simulink model "TPTC_Vehicle_dynamics_pedal2torque_NeglectSOC_R2024b"  (R2024b)
settings: Solver=ode23tb  StartTime=0.0  StopTime=40  RelTol=1e-3
model workspace (MAT data in the model file):
  BattChrgMax = -500000
  BattDischrgMax = 500000
  ChrgLmt_bpt = [1 1 1 1 1 1 1 1 0.7 0.35 0]
  DischrgLmt_bpt = [0 0.35 0.7 1 1 1 1 1 1 1 1]
  SOC_bpt = [0 10 20 30 40 50 60 70 80 90 100]
  motorMaxTorqueNm = [500 500 500 500 500 500 416.666666667 357.142857143 312.5 277.777777778 250 227.272727273 208.333333333 192.307692308 178.571428571 166.666666667]
  motorSpeedRadPs = [0 40 80 120 160 200 240 280 320 360 400 440 480 520 560 600]
undefined symbols (not defined in the file or in its folder): alpha_thr, dspblkCoreblockFVToolHelper, eta_drv, gcbh, gear_ratio_F, gear_ratio_R, J_axle, Kd_damp, R_tire, T_active, T_damp_lim, tau_lpf_damp, Tlim_down_rate, Tlim_up_rate, Tmax_mot, Ts_asr
libraries: autolibsharedcoupling x8, simulink x3, autolibshareddiff x2, autolibmappedmotor x2, slpidlib x1, autolibdatasheetbattery x1, sim3dlib x1, sim3dautolib x1, vehdynlibsteering x1
(part 1 of 3)
settings Model: Creator=jchu  LastModifiedBy=woaiw
settings ConfigComp: CovBoundaryAbsTol=1.0e-5

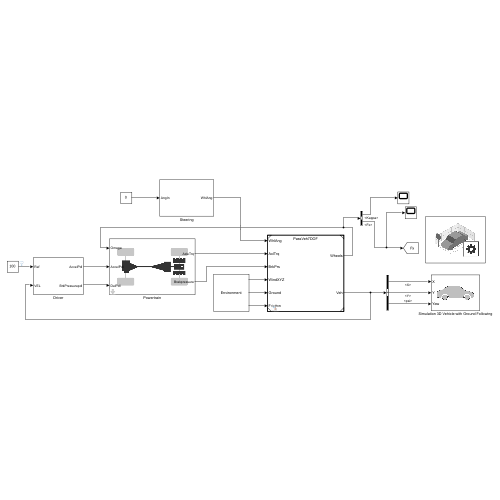
[thumbnail: Simulink's stored preview of the top-level diagram]
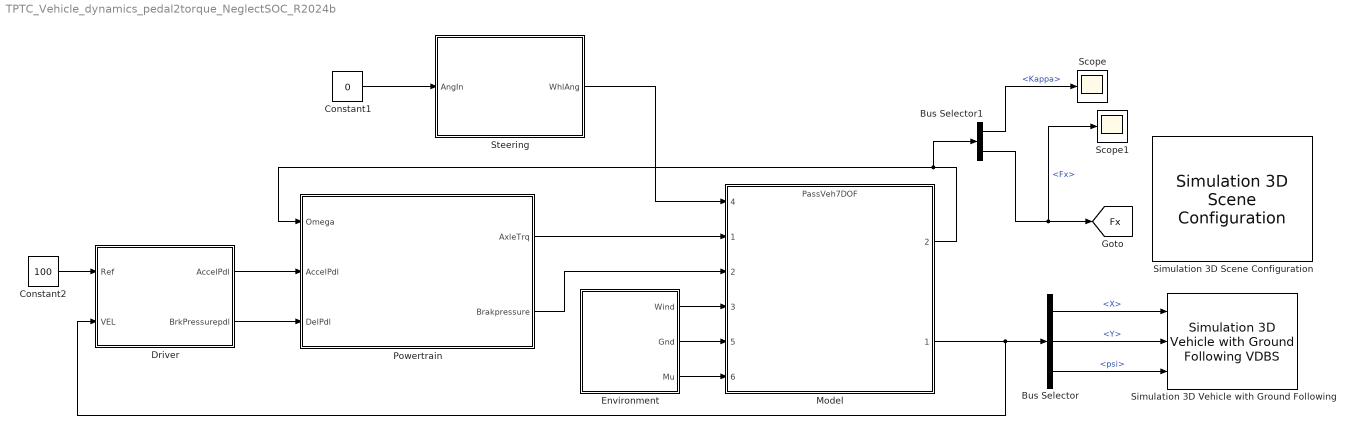
== system TPTC_Vehicle_dynamics_pedal2torque_NeglectSOC_R2024b ==
  Bus Selector : BusSelector  OutputSignals=InertFrm.Cg.Disp.X,InertFrm.Cg.Disp.Y,InertFrm.Cg.Ang.psi
  Bus Selector1 : BusSelector  OutputSignals=TireFrame.Kappa,TireFrame.Fx
  Constant1 : Constant  Value=0
  Constant2 : Constant  Value=100
  Driver : Subsystem
  Environment : Subsystem
      mask Display: disp('Environment')
  Model : ModelReference  ModelNameDialog=PassVeh7DOF.slx  SimulationMode=Normal  ModelReferenceVersion=9.3
      settings: PortSchema="{\"entries\":[{\"content\":{\"sides\":[{\"content\":{\"connectorIds\":[\"In4\",\"In1\",\"In2\",\"In3\",\"In5\",\"In6\"]},\"type\":\"ConnectorPlacement.EquallySpacedRectSide\",\"uuid\":\"e9709a47-3cb3-4a3a-94dc-e137fda36ac7\"},{\"content\":{\"connectorIds\":[\"Out2\",\"Out1\"],\"side\":\"RIGHT\"},\"type\":\"ConnectorPlacement.EquallySpacedRectSide\",\"uuid\":\"17c9465a-c7d2-47f9-932e-b722968c60f5\"},{\"content\":{\"side\":\"TOP\"},\"type\":\"ConnectorPlacement.EquallySpacedRectSide\",\"uuid\":\"38cd0d31-1510-4d7f-a224-4b6e7eb516ec\"}]},\"type\":\"ConnectorPlacement.EquallySpacedConnector\",\"uuid\":\"ef4f9ae8-cb52-4422-b25b-7a352d7601ce\"}],\"packageUris\":[\"http://schema.mathworks.com/mf0/Connector/R2020b\"],\"version\":\"1.0\"}"
  Powertrain : Subsystem
      mask DialogControl ParameterGroupVar Prompt: 参数
      mask Display: image('vdbslibpt.png');
  Scope : Scope
  Scope1 : Scope
  Simulation 3D Scene Configuration : sim3dlib/Simulation 3D Scene Configuration  Priority=0  ProjectFormat=Default Scenes  SceneDesc=Straight road  ProjectName=D:\Program Files\MATLAB\R2026a\toolbox\shared\sim3d_projects\automotive_project_windows\UE\WindowsNoEditor\VehicleSimulation.exe  ScenePath=/Game/Maps/HwStrght  EnableOpenDRIVE=off  vehTagList={'Custom';'Scene Origin';'SimulinkVehicle1'}  vehTag=SimulinkVehicle1  FreeCameraDefaultInitialTranslation=[-6, 0, 2]  FreeCameraDefaultInitialRotation=[0, -15, 0]  FreeCameraInitialTranslation=[0, 0, 0]  FreeCameraInitialRotation=[0, 0, 0]  OpVisEn=off  Ts=.02  EnableWindow=on  EnableRemoteAccess=off  SimulationMode=CoSimulation  SimulateUsing=Interpreted execution  EnableAnimationRecording=off  OverrideDefaultRecording=off  AnimationRecordingFileName=sim3dAnimation.mat  AnimationRecordingInterval=[0 inf]  EnableWeather=off  SunAzimuth=90  SunAltitude=40.0  EnableGeospatialSun=off  Latitude=0  Longitude=0  Date=2023-01-01  Time=10:30:00  GeoTimeZone=-5.0  SunDaylightSaving=off  wind=1  clouds=10  EnableVolumetricClouds=off  CloudCoverage=0  CloudAltitude=6  fog=0  rain=0  RaindropsEffect=off  SnowDensity=0  EnableGeospatial=off  UseTrueOrigin=off  OriginHeight=200  OriginLatitude=40.744652  OriginLongitude=-73.988864  MapStyle=Aerial  AdditionalAssetIDs=[]  UseAdvancedSunSky=off  SolarTime=11  TimeZone=-5  Day=21  Month=9  Year=2022  UseDaylightSavingTime=on  DSTStartDay=10  DSTStartMonth=3  DSTEndDay=3  DSTEndMonth=11  DSTSwitchHour=2  sensorTag=MainCamera1  sensorId=1  sensorName=MainCamera1  mountLoc=Origin  offsetFlag=off  tmountOffset=[0, 0, 0]  rmountOffset=[0, 0, 0]  HorizontalResolution=1280  VerticalResolution=720  HorizontalFOV=60  mountPoint=[0 0 0]  mountOrientation=[0 0 0]  aMode=2  ID=1  GeoTrigger=Inactive
      settings: LibrarySourceBlock=vehdynlibsim3dcore/Simulation 3D Scene Configuration
  Simulation 3D Vehicle with Ground Following : sim3dautolib/Simulation 3D Vehicle with Ground Following VDBS  Priority=-1  PassVehMesh=Muscle car  MeshPath=/MathWorksSimulation/Vehicles/Muscle/Meshes/SK_MuscleCar.SK_MuscleCar  TrackWidth=1.9  WheelBase=3  WheelRadius=0.35  VehColor=Red  InitialPos=[0, 0, 0]  InitialRot=[0, 0, 0]  ActorName=SimulinkVehicle1  VehLightsControl=off  HeadlightColor=[ 1, 1, 1 ]  HighBeamIntensity=100000  LowBeamIntensity=60000  HighBeamConeAngle=1.22  LowBeamConeAngle=1.22  LeftHeadlightOrientation=[ 0, 0 ]  RightHeadlightOrientation=[ 0, 0 ]  BrakelightIntensity=200  ReverselightIntensity=500  SignallightIntensity=500  SignallightPeriod=1  SignalPulseWidth=50  SampleTime=-1  ActorType=SimulinkVehicle  ID=1  aMode=2  ActorTag=SimulinkVehicle1  CoordinateScheme=SAE
      settings: LibrarySourceBlock=vehdynlibsim3d/Simulation 3D Vehicle with Ground Following
  Steering : Subsystem
  tag scope: Fx=global
  wires:
  Bus Selector/2 -> Simulation 3D Vehicle with Ground Following/2  "<Y>"
  Bus Selector/1 -> Simulation 3D Vehicle with Ground Following/1  "<X>"
  Bus Selector/3 -> Simulation 3D Vehicle with Ground Following/3  "<psi>"
  Environment/1(Wind) -> Model/3
  Environment/2(Gnd) -> Model/5
  Environment/3(Mu) -> Model/6
  Constant1/1 -> Steering/1(AngIn)
  Steering/1(WhlAng) -> Model/4
  Model/2 -> Bus Selector1/1, Powertrain/1(Omega)
  Powertrain/2(Brakpressure) -> Model/2
  Constant2/1 -> Driver/1(Ref)
  Model/1 -> Driver/2(VEL), Bus Selector/1
  Driver/1(AccelPdl) -> Powertrain/2(AccelPdl)
  Driver/2(BrkPressurepdl) -> Powertrain/3(DelPdl)
  Powertrain/1(AxleTrq) -> Model/1
  Bus Selector1/1 -> Scope/1  "<Kappa>"
  Bus Selector1/2 -> Scope1/1, [Fx]  "<Fx>"

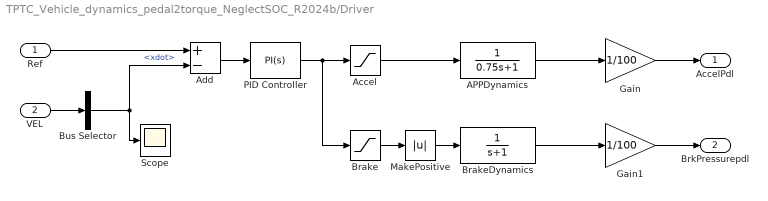
== system TPTC_Vehicle_dynamics_pedal2torque_NeglectSOC_R2024b/Driver ==
  Ref : Inport
  VEL : Inport  Port=2
  APPDynamics : TransferFcn  Denominator=[0.75 1]
  Accel : Saturate  UpperLimit=100  LowerLimit=0
  Add : Sum  Inputs=+-
  Brake : Saturate  UpperLimit=0  LowerLimit=-100
  BrakeDynamics : TransferFcn  Denominator=[1 1]
  Bus Selector : BusSelector  OutputSignals=BdyFrm.Cg.Vel.xdot
  Gain : Gain  Gain=1/100
  Gain1 : Gain  Gain=1/100
  MakePositive : Abs  SaturateOnIntegerOverflow=off
  PID Controller : slpidlib/PID Controller  Controller=PI  Form=Parallel  TimeDomain=Continuous-time  UseExternalTs=off  SampleTime=-1  IntegratorMethod=Forward Euler  FilterMethod=Forward Euler  ControllerParametersSource=internal  P=20  I=1  UseKiTs=off  D=0  UseExternalDerivativeSource=off  N=100  UseFilter=on  TunerSelectOption=Transfer Function Based (PID Tuner App)  InitialConditionSource=internal  InitialConditionForIntegrator=0  InitialConditionForFilter=0  DifferentiatorICPrevScaledInput=0  ExternalReset=none  TrackingMode=off  Kt=1  LimitOutput=on  SatLimitsSource=internal  UpperSaturationLimit=100  LowerSaturationLimit=-100  LinearizeAsGain=on  AntiWindupMode=none  Kb=1  LimitIntegrator=off  UpperIntegratorSaturationLimit=inf  LowerIntegratorSaturationLimit=-inf  POutMin=[]  POutMax=[]  IOutMin=[]  IOutMax=[]  DOutMin=[]  DOutMax=[]  NOutMin=[]  NOutMax=[]  SumOutMin=[]  SumOutMax=[]  SaturationOutMin=[]  SaturationOutMax=[]  PParamMin=[]  PParamMax=[]  IParamMin=[]  IParamMax=[]  DParamMin=[]  DParamMax=[]  NParamMin=[]  NParamMax=[]  KbParamMin=[]  KbParamMax=[]  KtParamMin=[]  KtParamMax=[]  KbOutMin=[]  KbOutMax=[]  KtOutMin=[]  KtOutMax=[]  IntegratorOutMin=[]  IntegratorOutMax=[]  FilterOutMin=[]  FilterOutMax=[]  SumI1OutMin=[]  SumI1OutMax=[]  SumI2OutMin=[]  SumI2OutMax=[]  SumI3OutMin=[]  SumI3OutMax=[]  SumI4OutMin=[]  SumI4OutMax=[]  SumDOutMin=[]  SumDOutMax=[]  DifferentiatorOutMin=[]  DifferentiatorOutMax=[]  FilterDiffOutCoefMin=[]  FilterDiffOutCoefMax=[]  ReciprocalOutMin=[]  ReciprocalOutMax=[]  SumDenOutMin=[]  SumDenOutMax=[]  SumNumOutMin=[]  SumNumOutMax=[]  DivideOutMin=[]  DivideOutMax=[]  UdiffTsProdOutMin=[]  UdiffTsProdOutMax=[]  NTsProdOutMin=[]  NTsProdOutMax=[]  UintegralTsProdOutMin=[]  UintegralTsProdOutMax=[]  UngainTsProdOutMin=[]  UngainTsProdOutMax=[]  ClampingZeroOutDataTypeStr=Inherit: Inherit via back propagation  ClampingZeroOutMin=[]  ClampingZeroOutMax=[]  FilterDenConstantOutDataTypeStr=Inherit: Inherit via back propagation  FilterDenConstantOutMin=[]  FilterDenConstantOutMax=[]  PCopyOutDataTypeStr=Inherit: Inherit via back propagation  PCopyOutMin=[]  PCopyOutMax=[]  NCopyOutDataTypeStr=Inherit: Inherit via back propagation  NCopyOutMin=[]  NCopyOutMax=[]  IntegratorContinuousStateAttributes=''  IntegratorStateMustResolveToSignalObject=off  IntegratorRTWStateStorageClass=Auto  FilterContinuousStateAttributes=''  FilterStateMustResolveToSignalObject=off  FilterRTWStateStorageClass=Auto  ParallelPVariant=InternalParameters  IdealPVariant=Disabled  IVariant=InternalParameters  DVariant=Disabled  IntegratorVariant=Continuous  SatVariant=Enabled  AWVariant=Passthrough  PCopyVariant=Disabled  TRVariant=Disabled  FdbkBlocksVariant=Forward  IdealPFdbkVariant=Disabled  SatFdbkVariant=Disabled  DerivativeFilterVariant=Disabled  NVariant=Disabled  NCopyVariant=Disabled_SignalSpec  FilterICVariant=Disabled  IntegratorICVariant=InternalICs  ExternalResetVariant=Disabled  TRSumVariant=Passthrough  SumFdbkVariant=Disabled  SumVariant=Sum_PI  TsampFilterVariant=InternalTs  TsampNgainVariant=Passthrough  TsampIntegralVariant=Disabled_SignalSpec  ExternalSaturationOutDataTypeStr=Inherit: Same as second input  DerivativeSourceVariant=Disabled  PreIntVariant=InternalPreInt
  Scope : Scope
  AccelPdl : Outport
  BrkPressurepdl : Outport  Port=2
  wires:
  APPDynamics/1 -> Gain/1
  PID Controller/1 -> Accel/1, Brake/1
  MakePositive/1 -> BrakeDynamics/1
  Accel/1 -> APPDynamics/1
  Add/1 -> PID Controller/1
  Brake/1 -> MakePositive/1
  Ref/1 -> Add/1
  BrakeDynamics/1 -> Gain1/1
  Gain/1 -> AccelPdl/1
  Gain1/1 -> BrkPressurepdl/1
  VEL/1 -> Bus Selector/1
  Bus Selector/1 -> Scope/1, Add/2  "<xdot>"

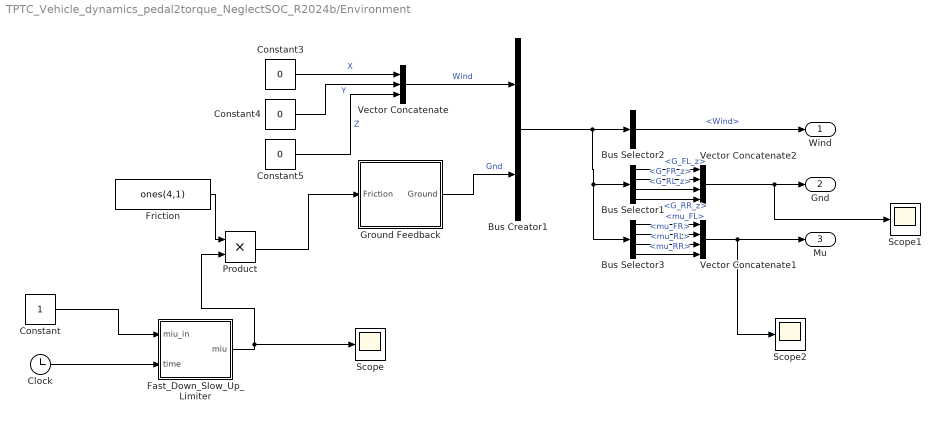
== system TPTC_Vehicle_dynamics_pedal2torque_NeglectSOC_R2024b/Environment ==
  Bus Creator1 : BusCreator  Inputs=2
  Bus Selector1 : BusSelector  OutputSignals=Gnd.z.G_FL_z,Gnd.z.G_FR_z,Gnd.z.G_RL_z,Gnd.z.G_RR_z
  Bus Selector2 : BusSelector  OutputSignals=Wind
  Bus Selector3 : BusSelector  OutputSignals=Gnd.mu.mu_FL,Gnd.mu.mu_FR,Gnd.mu.mu_RL,Gnd.mu.mu_RR
  Clock : Clock
  Constant : Constant
  Constant3 : Constant  Value=0
  Constant4 : Constant  Value=0
  Constant5 : Constant  Value=0
  Fast_Down_Slow_Up_Limiter : MATLAB Function  TreatAsAtomicUnit=on  SystemSampleTime=Ts_asr
  Friction : Constant  Value=ones(4,1)
  Ground Feedback : Subsystem  Variant=on  VariantControlMode=label  LabelModeActiveChoice=0
  Product : Product
  Scope : Scope
  Scope1 : Scope
  Scope2 : Scope
  Vector Concatenate : Concatenate  NumInputs=3
  Vector Concatenate1 : Concatenate  NumInputs=4
  Vector Concatenate2 : Concatenate  NumInputs=4
  Wind : Outport
  Gnd : Outport  Port=2
  Mu : Outport  Port=3
  wires:
  Constant5/1 -> Vector Concatenate/3  "Z"
  Vector Concatenate/1 -> Bus Creator1/1  "Wind"
  Constant3/1 -> Vector Concatenate/1  "X"
  Constant4/1 -> Vector Concatenate/2  "Y"
  Ground Feedback/1(Ground) -> Bus Creator1/2  "Gnd"
  Friction/1 -> Product/1
  Bus Selector3/1 -> Vector Concatenate1/1  "<mu_FL>"
  Vector Concatenate1/1 -> Scope2/1, Mu/1
  Bus Selector2/1 -> Wind/1  "<Wind>"
  Vector Concatenate2/1 -> Scope1/1, Gnd/1
  Bus Selector3/3 -> Vector Concatenate1/3  "<mu_RL>"
  Bus Selector3/4 -> Vector Concatenate1/4  "<mu_RR>"
  Bus Selector1/2 -> Vector Concatenate2/2  "<G_FR_z>"
  Bus Creator1/1 -> Bus Selector3/1, Bus Selector1/1, Bus Selector2/1
  Bus Selector3/2 -> Vector Concatenate1/2  "<mu_FR>"
  Bus Selector1/4 -> Vector Concatenate2/4  "<G_RR_z>"
  Bus Selector1/1 -> Vector Concatenate2/1  "<G_FL_z>"
  Bus Selector1/3 -> Vector Concatenate2/3  "<G_RL_z>"
  Product/1 -> Ground Feedback/1(Friction)
  Clock/1 -> Fast_Down_Slow_Up_Limiter/2(time)
  Constant/1 -> Fast_Down_Slow_Up_Limiter/1(miu_in)
  Fast_Down_Slow_Up_Limiter/1(miu) -> Product/2, Scope/1

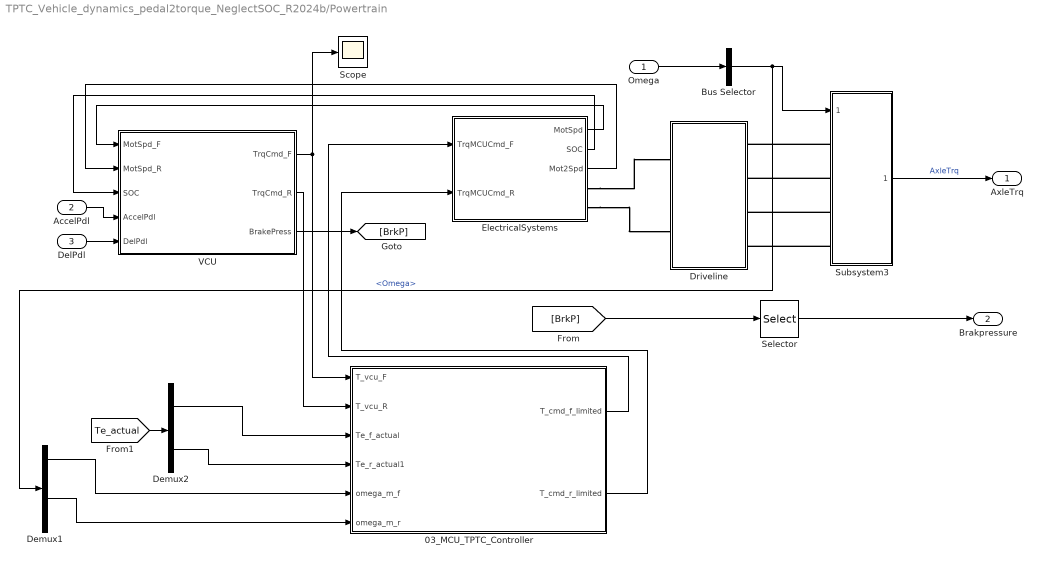
== system TPTC_Vehicle_dynamics_pedal2torque_NeglectSOC_R2024b/Powertrain ==
  Omega : Inport
  AccelPdl : Inport  Port=2
  DelPdl : Inport  Port=3
  03_MCU_TPTC_Controller : Subsystem
  Bus Selector : BusSelector  OutputSignals=TireFrame.Omega
  Demux1 : Demux
  Demux2 : Demux  Outputs=2
  Driveline : Subsystem
  ElectricalSystems : Subsystem
  Scope : Scope
  Selector : Selector  InputPortWidth=1  IndexOptions=Index vector (dialog)  Indices=[1 1 1 1]  OutputSizes=1
  Subsystem3 : Subsystem
  VCU : Subsystem
  AxleTrq : Outport
  Brakpressure : Outport  Port=2
  wires:
  ElectricalSystems/2(SOC) -> VCU/3(SOC)
  Subsystem3/1(AxleTrq) -> AxleTrq/1  "AxleTrq"
  AccelPdl/1 -> VCU/4(AccelPdl)
  Omega/1 -> Bus Selector/1
  Bus Selector/1 -> Demux1/1, Subsystem3/1(WhlSpd)  "<Omega>"
  ElectricalSystems/1(MotSpd) -> VCU/1(MotSpd_F)
  VCU/3(BrakePress) -> [BrkP]
  DelPdl/1 -> VCU/5(DelPdl)
  Selector/1 -> Brakpressure/1
  [BrkP] -> Selector/1
  VCU/1(TrqCmd_F) -> Scope/1, 03_MCU_TPTC_Controller/1(T_vcu_F)
  VCU/2(TrqCmd_R) -> 03_MCU_TPTC_Controller/2(T_vcu_R)
  03_MCU_TPTC_Controller/1("T_cmd_f_limited  ") -> ElectricalSystems/1(TrqMCUCmd_F)
  03_MCU_TPTC_Controller/2("T_cmd_r_limited ") -> ElectricalSystems/2(TrqMCUCmd_R)
  Demux1/3 -> 03_MCU_TPTC_Controller/6(omega_m_r)
  Demux1/1 -> 03_MCU_TPTC_Controller/5(omega_m_f)
  Demux2/1 -> 03_MCU_TPTC_Controller/3(Te_f_actual)
  Demux2/2 -> 03_MCU_TPTC_Controller/4(Te_r_actual1)
  ElectricalSystems/3(Mot2Spd) -> VCU/2(MotSpd_R)
  [Te_actual] -> Demux2/1
  connections:
  Subsystem3/LConn1 -- Driveline/RConn1
  ElectricalSystems/RConn1 -- Driveline/LConn1
  Subsystem3/LConn2 -- Driveline/RConn2
  Subsystem3/LConn3 -- Driveline/RConn3
  Subsystem3/LConn4 -- Driveline/RConn4
  ElectricalSystems/RConn2 -- Driveline/LConn2

== system TPTC_Vehicle_dynamics_pedal2torque_NeglectSOC_R2024b/Steering ==
  AngIn : Inport
  Ground1 : Ground
  Ground2 : Ground
  Kinematic Steering : vehdynlibsteering/Kinematic Steering  StrgType=Rack and pinion  StrgRatioType=Constant  Loc=Front  NrmlFctr=0.01  TrckWdth=1  WhlBase=1.524  Db=0  StrgRng=1.25*pi  StrgAngBpts="[-6.2832   -5.0265   -3.7699   -2.5133   -1.2566         0    1.2566    2.5133    3.7699    5.0265    6.2832]"  StrgRatioTbl=|  StrgRatio=100  PctAckIn=off  PctAck=100  PctAckTbl=ones(1,11)*100  StrgArmLngth=0.1  RckCsLngth=0.5  TieRodLngth=0.248  D=0.2  PnnRadius=0.00085818  PnnRadiusTbl="[0.0055    0.0055    0.0056    0.0057    0.0058    0.0057    0.0057    0.0057    0.0056    0.0055    0.0055]"  RodLngth=0.1  ParaArmLngth=0.9  aMode=2
      | [13.5000   13.3750   13.2500   13.1250   13.0000   13.0000   13.0000   13.1250   13.2500   13.3750   13.5000
      | ]
  Mux : Mux
  WhlAng : Outport
  wires:
  Kinematic Steering/3 -> Mux/2
  Ground1/1 -> Mux/3
  Ground2/1 -> Mux/4
  Kinematic Steering/2 -> Mux/1
  Mux/1 -> WhlAng/1
  AngIn/1 -> Kinematic Steering/1

== system TPTC_Vehicle_dynamics_pedal2torque_NeglectSOC_R2024b/Environment/Ground Feedback ==
  Friction : Inport
  Constant : Subsystem  VariantControl=0
  Ground : Outport  VectorParamsAs1DForOutWhenUnconnected=off

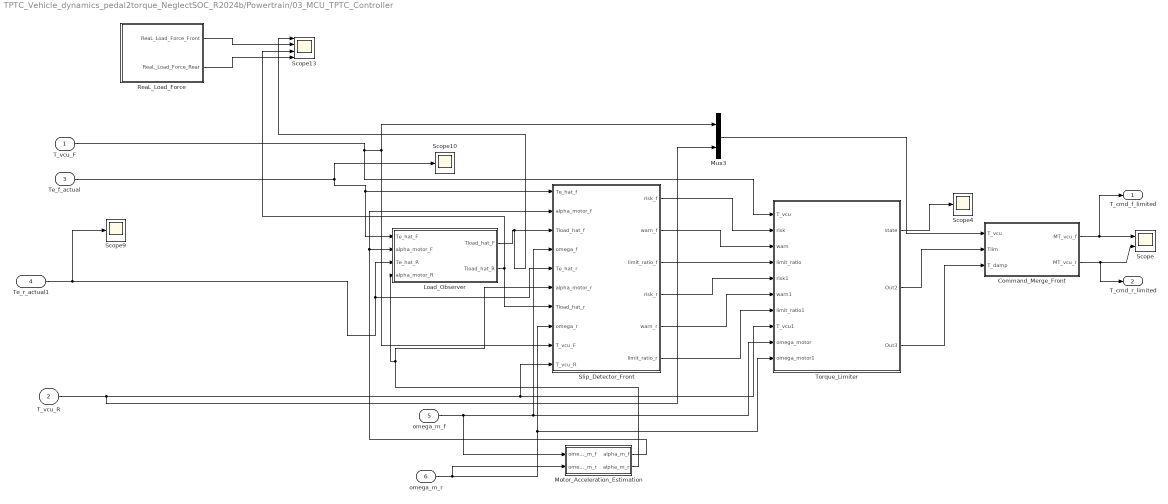
== system TPTC_Vehicle_dynamics_pedal2torque_NeglectSOC_R2024b/Powertrain/03_MCU_TPTC_Controller ==
  T_vcu_F : Inport
  T_vcu_R : Inport  Port=2
  Te_f_actual : Inport  Port=3
  Te_r_actual1 : Inport  Port=4
  omega_m_f : Inport  Port=5
  omega_m_r : Inport  Port=6
  Command_Merge_Front : Subsystem
  Load_Observer : Subsystem
  Motor_Acceleration_Estimation : Subsystem
  Mux3 : Mux  Inputs=2
  ReaL_Load_Force : Subsystem
  Scope : Scope  NumInputPorts=2
  Scope10 : Scope
  Scope13 : Scope  NumInputPorts=4
  Scope4 : Scope
  Scope9 : Scope
  Slip_Detector_Front : Subsystem
  Torque_Limiter : Subsystem
  "T_cmd_f_limited  " : Outport
  "T_cmd_r_limited " : Outport  Port=2
  wires:
  Motor_Acceleration_Estimation/2(alpha_m_r) -> Slip_Detector_Front/6(alpha_motor_r), Load_Observer/4(alpha_motor_R)
  Motor_Acceleration_Estimation/1(alpha_m_f) -> Slip_Detector_Front/2(alpha_motor_f), Load_Observer/2(alpha_motor_F)
  omega_m_r/1 -> Motor_Acceleration_Estimation/2(omega_m_r), Torque_Limiter/10(omega_motor1), Slip_Detector_Front/8(omega_r)
  Mux3/1 -> Command_Merge_Front/1(T_vcu)
  Command_Merge_Front/1(MT_vcu_f) -> "T_cmd_f_limited  "/1, Scope/1
  Command_Merge_Front/2(MT_vcu_r) -> Scope/2, "T_cmd_r_limited "/1
  Te_f_actual/1 -> Load_Observer/1(Te_hat_F), Slip_Detector_Front/1(Te_hat_f), Scope10/1
  Te_r_actual1/1 -> Scope9/1, Load_Observer/3(Te_hat_R), Slip_Detector_Front/5(Te_hat_r)
  T_vcu_R/1 -> Mux3/2, Torque_Limiter/8(T_vcu1), Slip_Detector_Front/10(T_vcu_R)
  omega_m_f/1 -> Motor_Acceleration_Estimation/1(omega_m_f), Torque_Limiter/9(omega_motor), Slip_Detector_Front/4(omega_f)
  T_vcu_F/1 -> Torque_Limiter/1(T_vcu), Slip_Detector_Front/9(T_vcu_F), Mux3/1
  Load_Observer/1(Tload_hat_F) -> Scope13/1, Slip_Detector_Front/3(Tload_hat_f)
  ReaL_Load_Force/1(ReaL_Load_Force_Front) -> Scope13/2
  ReaL_Load_Force/2(ReaL_Load_Force_Rear) -> Scope13/4
  Load_Observer/2(Tload_hat_R) -> Scope13/3, Slip_Detector_Front/7(Tload_hat_r)
  Slip_Detector_Front/1(risk_f) -> Torque_Limiter/2(risk)
  Slip_Detector_Front/2(warn_f) -> Torque_Limiter/3(warn)
  Slip_Detector_Front/3(limit_ratio_f) -> Torque_Limiter/4(limit_ratio)
  Slip_Detector_Front/4(risk_r) -> Torque_Limiter/5(risk1)
  Slip_Detector_Front/5(warn_r) -> Torque_Limiter/6(warn1)
  Slip_Detector_Front/6(limit_ratio_r) -> Torque_Limiter/7(limit_ratio1)
  Torque_Limiter/1(state) -> Scope4/1
  Torque_Limiter/2(Out2) -> Command_Merge_Front/2(Tlim)
  Torque_Limiter/3(Out3) -> Command_Merge_Front/3(T_damp)

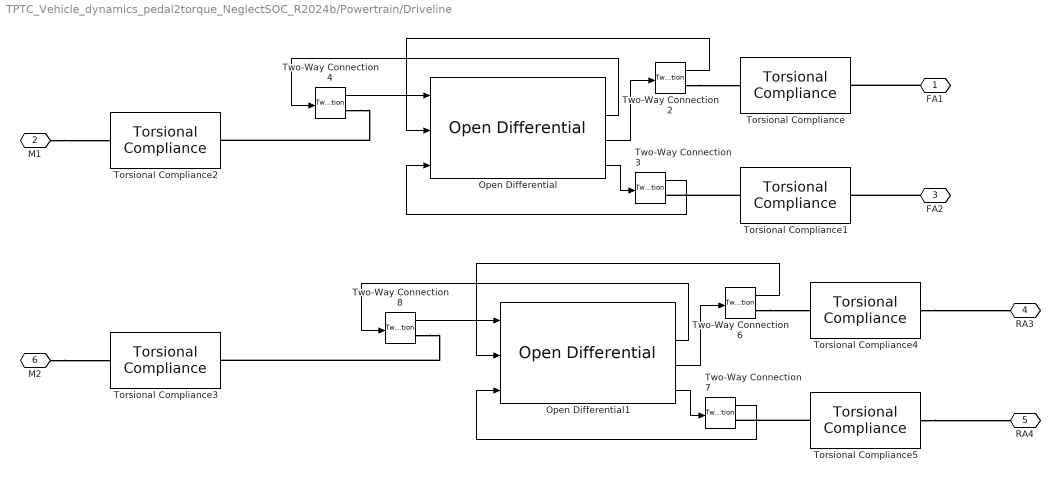
== system TPTC_Vehicle_dynamics_pedal2torque_NeglectSOC_R2024b/Powertrain/Driveline ==
  Open Differential : autolibshareddiff/Open Differential  DiffEffModelPopup=Constant  InterpMethod=Linear point-slope  extTamb=off  shaftSwitchMask=To the left of center-line  Ndiff=10.91  Jd=.1  bd=1e-3  Jw1=0.019  bw1=1e-3  Jw2=0.019  bw2=1e-3  omegaw1o=0  omegaw2o=0  eta=1  eta_tbl=reshape([0.64 0.76 0.8 0.81 0.83 0.84 0.84 0.56 0.73 0.78 0.8 0.83 0.84 0.84 0.54 0.71 0.77 0.8 0.82 0.84 0.84 0.53 0.71 0.77 0.8 0.83 0.84 0.84 0.51 0.71 0.77 0.8 0.83 0.84 0.85 0.52 0.7 0.77 0.8 0.83 0.84 0.85 0.51 0.71 0.76 0.79 0.83 0.84 0.85 0.5 0.69 0.76 0.79 0.82 0.84 0.85 0.45 0.68 0.75 0.78 0.82 0.84 0.85 0.43 0.67 0.74 0.78 0.81 0.83 0.84 0.38 0.63 0.71 0.75 0.8 0.82 0.83 0.81 0.86 0.88 0.89 0.89 0.89 0.9 0.77 0.85 0.87 0.88 0.89 0.9 0.9 0.72 0.82 0.86 0.87 0.88 0.89 0.9 0.68 0.8 0.84 0.86 0.88 0.89 0.89 0.67 0.8 0.84 0.86 0.88 0.89 0.9 0.67 0.8 0.84 0.86 0.88 0.89 0.9 0.65 0.8 0.84 0.86 0.88 0.89 0.9 0.64 0.79 0.83 0.86 0.88 0.89 0.9 0.63 0.78 0.83 0.86 0.88 0.89 0.9 0.59 0.76 0.82 0.85 0.87 0.89 0.9 0.53 0.73 0.8 0.83 0.86 0.88 0.89], 7, 11, 2)  Trq_bpts=[25, 50, 75, 100, 150, 200, 250]  omega_bpts=[52.4 78.5 105 131 157 183 209 262 314 419 524]  Temp_bpts=[290 358]  Tamb=297.15  maxAbsSpd=5e3  aMode=1
      settings: LibrarySourceBlock=autolibdiff/Open Differential
  Open Differential1 : autolibshareddiff/Open Differential  DiffEffModelPopup=Constant  InterpMethod=Linear point-slope  extTamb=off  shaftSwitchMask=To the left of center-line  Ndiff=11.62  Jd=.1  bd=1e-3  Jw1=0.016  bw1=1e-3  Jw2=0.016  bw2=1e-3  omegaw1o=0  omegaw2o=0  eta=1  eta_tbl=reshape([0.64 0.76 0.8 0.81 0.83 0.84 0.84 0.56 0.73 0.78 0.8 0.83 0.84 0.84 0.54 0.71 0.77 0.8 0.82 0.84 0.84 0.53 0.71 0.77 0.8 0.83 0.84 0.84 0.51 0.71 0.77 0.8 0.83 0.84 0.85 0.52 0.7 0.77 0.8 0.83 0.84 0.85 0.51 0.71 0.76 0.79 0.83 0.84 0.85 0.5 0.69 0.76 0.79 0.82 0.84 0.85 0.45 0.68 0.75 0.78 0.82 0.84 0.85 0.43 0.67 0.74 0.78 0.81 0.83 0.84 0.38 0.63 0.71 0.75 0.8 0.82 0.83 0.81 0.86 0.88 0.89 0.89 0.89 0.9 0.77 0.85 0.87 0.88 0.89 0.9 0.9 0.72 0.82 0.86 0.87 0.88 0.89 0.9 0.68 0.8 0.84 0.86 0.88 0.89 0.89 0.67 0.8 0.84 0.86 0.88 0.89 0.9 0.67 0.8 0.84 0.86 0.88 0.89 0.9 0.65 0.8 0.84 0.86 0.88 0.89 0.9 0.64 0.79 0.83 0.86 0.88 0.89 0.9 0.63 0.78 0.83 0.86 0.88 0.89 0.9 0.59 0.76 0.82 0.85 0.87 0.89 0.9 0.53 0.73 0.8 0.83 0.86 0.88 0.89], 7, 11, 2)  Trq_bpts=[25, 50, 75, 100, 150, 200, 250]  omega_bpts=[52.4 78.5 105 131 157 183 209 262 314 419 524]  Temp_bpts=[290 358]  Tamb=297.15  maxAbsSpd=5e3  aMode=1
      settings: LibrarySourceBlock=autolibdiff/Open Differential
  Torsional Compliance{,1..5} (6 alike) : autolibsharedcoupling/Torsional Compliance  port_config=Two-way connection  extInfo=off  k=1e4  b=1e2  theta_o=0  domega_o=0  omega_c=3000  blkID=0  aMode=1
  Two-Way Connection{2..4,6..8} (6 alike) : TwoWayConnection
  FA1 : PMIOPort  Side=Right
  M1 : PMIOPort  Port=2  Side=Left
  FA2 : PMIOPort  Port=3  Side=Right
  RA3 : PMIOPort  Port=4  Side=Right
  RA4 : PMIOPort  Port=5  Side=Right
  M2 : PMIOPort  Port=6  Side=Left
  wires:
  Two-Way Connection3/1 -> Open Differential/3
  Two-Way Connection2/1 -> Open Differential/2
  Open Differential/4 -> Two-Way Connection3/1
  Open Differential/2 -> Two-Way Connection4/1
  Two-Way Connection4/1 -> Open Differential/1
  Open Differential/3 -> Two-Way Connection2/1
  Two-Way Connection8/1 -> Open Differential1/1
  Open Differential1/3 -> Two-Way Connection6/1
  Two-Way Connection6/1 -> Open Differential1/2
  Two-Way Connection7/1 -> Open Differential1/3
  Open Differential1/2 -> Two-Way Connection8/1
  Open Differential1/4 -> Two-Way Connection7/1
  connections:
  Two-Way Connection2/RConn1 -- Torsional Compliance/LConn1
  M1/RConn1 -- Torsional Compliance2/LConn1
  Two-Way Connection4/RConn1 -- Torsional Compliance2/RConn1
  Torsional Compliance1/LConn1 -- Two-Way Connection3/RConn1
  FA1/RConn1 -- Torsional Compliance/RConn1
  FA2/RConn1 -- Torsional Compliance1/RConn1
  M2/RConn1 -- Torsional Compliance3/LConn1
  Two-Way Connection6/RConn1 -- Torsional Compliance4/LConn1
  Torsional Compliance5/LConn1 -- Two-Way Connection7/RConn1
  Torsional Compliance4/RConn1 -- RA3/RConn1
  Torsional Compliance5/RConn1 -- RA4/RConn1
  Two-Way Connection8/RConn1 -- Torsional Compliance3/RConn1

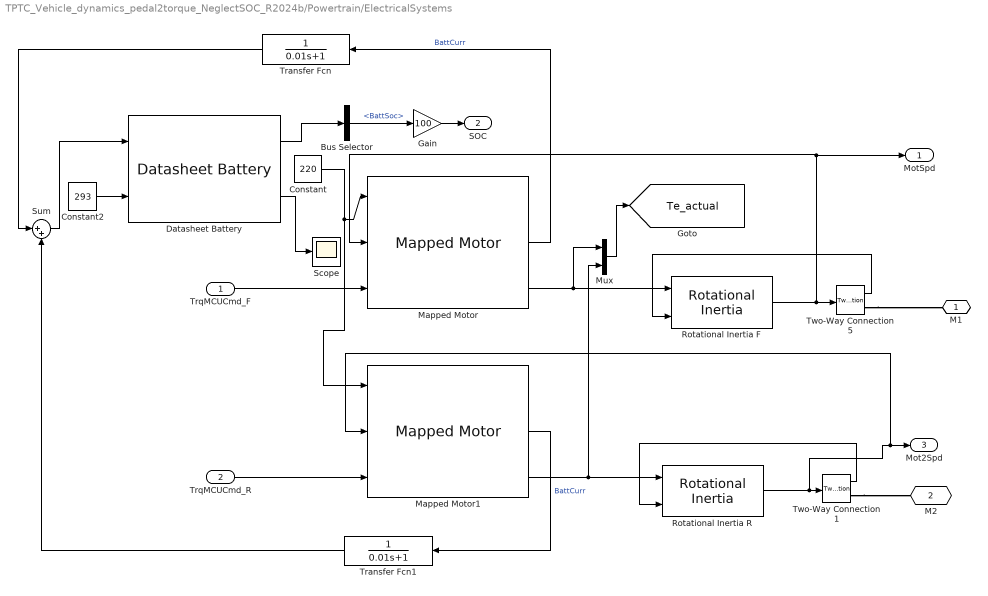
== system TPTC_Vehicle_dynamics_pedal2torque_NeglectSOC_R2024b/Powertrain/ElectricalSystems ==
  TrqMCUCmd_F : Inport
  TrqMCUCmd_R : Inport  Port=2
  Bus Selector : BusSelector  OutputSignals=BattSoc
  Constant : Constant  Value=220
  Constant2 : Constant  Value=293
  Datasheet Battery : autolibdatasheetbattery/Datasheet Battery  CapacityCtrl=Parameter  OutputVlt=Unfiltered  BattChargeMax=100  Em=[2.8 3.228 3.284 3.361 3.408 3.427 3.472 3.477 3.493 3.504 3.516 3.528 3.537 3.545 3.555 3.561 3.566 3.576 3.587 3.589 3.594 3.6 3.608 3.61 3.616 3.619 3.626 3.632 3.637 3.64 3.645 3.646 3.652 3.655 3.658 3.661 3.664 3.668 3.673 3.678 3.68 3.681 3.686 3.692 3.699 3.702 3.705 3.71 3.717 3.723 3.728 3.733 3.735 3.742 3.749 3.755 3.761 3.768 3.773 3.78 3.791 3.798 3.798 3.814 3.818 3.825 3.841 3.846 3.855 3.863 3.877 3.885 3.894 3.907 3.919 3.926 3.935 3.944 3.954 3.964 3.974 3.988 3.998 4.014 4.029 4.034 4.047 4.065 4.074 4.086 4.097 4.131 4.126 4.138 4.15 4.18 4.174 4.187 4.207 4.231 4.221]  CapLUTBp=[0 0.01 0.02 0.03 0.04 0.05 0.06 0.07 0.08 0.09 0.1 0.11 0.12 0.13 0.14 0.15 0.16 0.17 0.18 0.19 0.2 0.21 0.22 0.23 0.24 0.25 0.26 0.27 0.28 0.29 0.3 0.31 0.32 0.33 0.34 0.35 0.36 0.37 0.38 0.39 0.4 0.41 0.42 0.43 0.44 0.45 0.46 0.47 0.48 0.49 0.5 0.51 0.52 0.53 0.54 0.55 0.56 0.57 0.58 0.59 0.6 0.61 0.62 0.63 0.64 0.65 0.66 0.67 0.68 0.69 0.7 0.71 0.72 0.73 0.74 0.75 0.76 0.77 0.78 0.79 0.8 0.81 0.82 0.83 0.84 0.85 0.86 0.87 0.88 0.89 0.9 0.91 0.92 0.93 0.94 0.95 0.96 0.97 0.98 0.99 1]  RInt=[0.008846 0.009319 0.009027 0.00847 0.01032 0.01314;0.006389 0.006554 0.005553 0.005525 0.006043 0.007805;0.004364 0.004101 0.00406 0.003452 0.003846 0.004517;0.002031 0.002563 0.002532 0.00246 0.002716 0.003047;0.001443 0.001825 0.001795 0.001778 0.001924 0.002234;0.0005603 0.0007192 0.0006887 0.0007557 0.0007355 0.001014;0.001028 0.001338 0.001 0.001536 0.001546 0.002789]  BattTempBp=[243.1 253.1 263.1 273.1 283.1 298.1 313.1]  CapSOCBp=[0 0.2 0.4 0.6 0.8 1]  Ns=30  Np=2  BattCapInit=60  Tc=1/1000  Vinit=4.221  RefBlkName='autolibdatasheetbattery/Datasheet Battery'
  Gain : Gain  Gain=100
  Mapped Motor : autolibmappedmotor/Mapped Motor  w_Tmax_bp_ext=w_Tmax_bp  Tmax_w_V_ext=Tmax_w_V  w_Tmin_bp_ext=w_Tmin_bp  Tmin_w_V_ext=Tmin_w_V  port_config=Speed  param_by=Tabulated torque-speed envelope  w_t=motorSpeedRadPs  T_t=motorMaxTorqueNm  torque_max=.1  power_max=30  SpreadsheetTqLimitsFileName=MotorCalibrationImportData.xlsx  Tmax_w_V=[0.09 0.09 0.09;0.08 0.08 0.08;0.07 0.07 0.07;0 0 0]  w_Tmax_bp=[ 0 375 750 800 ]  V_Tmax_bp=[500 750 900]  Tmin_w_V=[-0.09 -0.09 -0.09;-0.08 -0.08 -0.08;-0.07 -0.07 -0.07;0 0 0]  w_Tmin_bp=[ 0 375 750 800 ]  V_Tmin_bp=[500 750 900]  Tc=0.02  param_loss=Single efficiency measurement  SpreadsheetLossFileName=MotorCalibrationImportData.xlsx  SpreadsheetEffFileName=MotorCalibrationImportData.xlsx  eff=100  w_eff=375  T_eff=0.08  Piron=0  Pbase=0  w_eff_bp=[-8000 -4000 0 4000 8000]  T_eff_bp=[0 0.03 0.06 0.09]  Temp_eff_bp=[233.15 293.15 373.15]  V_eff_bp=[500 700 900]  losses_table=[1.49 1.67 2.21 3.10; 0.42 0.69 1.14 2.03; 0.06 0.24 0.78 1.68; 0.42 0.69 1.14 2.03; 1.49 1.67 2.21 3.10]  losses_table_3d=cat(3,1.05*[1.49 1.67 2.21 3.10; 0.42 0.69 1.14 2.03; 0.06 0.24 0.78 1.68; 0.42 0.69 1.14 2.03; 1.49 1.67 2.21 3.10],[1.49 1.67 2.21 3.10; 0.42 0.69 1.14 2.03; 0.06 0.24 0.78 1.68; 0.42 0.69 1.14 2.03; 1.49 1.67 2.21 3.10],1.03*[1.49 1.67 2.21 3.10; 0.42 0.69 1.14 2.03; 0.06 0.24 0.78 1.68; 0.42 0.69 1.14 2.03; 1.49 1.67 2.21 3.10])  losses_table_4d=cat(4,cat(3,[1.5645 0.441 0.063 0.441 1.5645;1.7535 0.7245 0.252 0.7245 1.7535;2.3205 1.197 0.819 1.197 2.3205;3.255 2.1315 1.764 2.1315 3.255],[1.5645 0.441 0.063 0.441 1.5645;1.7535 0.7245 0.252 0.7245 1.7535;2.3205 1.197 0.819 1.197 2.3205;3.255 2.1315 1.764 2.1315 3.255],[1.5645 0.441 0.063 0.441 1.5645;1.7535 0.7245 0.252 0.7245 1.7535;2.3205 1.197 0.819 1.197 2.3205;3.255 2.1315 1.764 2.1315 3.255]),cat(3,[1.49 0.42 0.06 0.42 1.49;1.67 0.69 0.24 0.69 1.67;2.21 1.14 0.78 1.14 2.21;3.1 2.03 1.68 2.03 3.1],[1.49 0.42 0.06 0.42 1.49;1.67 0.69 0.24 0.69 1.67;2.21 1.14 0.78 1.14 2.21;3.1 2.03 1.68 2.03 3.1],[1.49 0.42 0.06 0.42 1.49;1.67 0.69 0.24 0.69 1.67;2.21 1.14 0.78 1.14 2.21;3.1 2.03 1.68 2.03 3.1]),cat(3,[1.5347 0.4326 0.0618 0.4326 1.5347;1.7201 0.7107 0.2472 0.7107 1.7201;2.2763 1.1742 0.8034 1.1742 2.2763;3.193 2.0909 1.7304 2.0909 3.193],[1.5347 0.4326 0.0618 0.4326 1.5347;1.7201 0.7107 0.2472 0.7107 1.7201;2.2763 1.1742 0.8034 1.1742 2.2763;3.193 2.0909 1.7304 2.0909 3.193],[1.5347 0.4326 0.0618 0.4326 1.5347;1.7201 0.7107 0.2472 0.7107 1.7201;2.2763 1.1742 0.8034 1.1742 2.2763;3.193 2.0909 1.7304 2.0909 3.193]))  efficiency_table=[95 95 95 95; 95 95 95 95; 95 95 95 95; 95 95 95 95; 95 95 95 95]  efficiency_table_3d=cat(3,90*ones(5,4),95*ones(5,4),92*ones(5,4))  efficiency_table_4d=cat(4,cat(3,90*ones(5,4)',90*ones(5,4)',90*ones(5,4)'),cat(3,95*ones(5,4)',95*ones(5,4)',95*ones(5,4)'),cat(3,92*ones(5,4)',92*ones(5,4)',92*ones(5,4)'))  J=5e-6  b=1e-5  omega_o=0  T_t_extended=[166.666666666667 178.571428571429 192.307692307692 208.333333333333 227.272727272727 250 277.777777777778 312.5 357.142857142857 416.666666666667 500 500 500 500 500 500 500 500 500 500 500 416.666666666667 357.142857142857 312.5 277.777777777778 250 227.272727272727 208.333333333333 192.307692307692 178.571428571429 166.666666666667]  w_t_extended=[-600 -560 -520 -480 -440 -400 -360 -320 -280 -240 -200 -160 -120 -80 -40 0 40 80 120 160 200 240 280 320 360 400 440 480 520 560 600]  KLossIron=0  KLossCopper=0  x_w_eff_vec=[-8000 -4000 0 4000 8000]  x_T_eff_vec=[-0.09 -0.06 -0.03 0 0.03 0.06 0.09]  x_tmp_eff_vec=[233.15 293.15 373.15]  x_V_eff_vec=[500 700 900]  x_losses_mat=[3.1 2.21 1.67 1.49 1.67 2.21 3.1;2.03 1.14 0.69 0.42 0.69 1.14 2.03;1.68 0.78 0.24 0.06 0.24 0.78 1.68;2.03 1.14 0.69 0.42 0.69 1.14 2.03;3.1 2.21 1.67 1.49 1.67 2.21 3.1]  x_losses_mat_3d=cat(3,[3.255 2.3205 1.7535 1.5645 1.7535 2.3205 3.255;2.1315 1.197 0.7245 0.441 0.7245 1.197 2.1315;1.764 0.819 0.252 0.063 0.252 0.819 1.764;2.1315 1.197 0.7245 0.441 0.7245 1.197 2.1315;3.255 2.3205 1.7535 1.5645 1.7535 2.3205 3.255],[3.1 2.21 1.67 1.49 1.67 2.21 3.1;2.03 1.14 0.69 0.42 0.69 1.14 2.03;1.68 0.78 0.24 0.06 0.24 0.78 1.68;2.03 1.14 0.69 0.42 0.69 1.14 2.03;3.1 2.21 1.67 1.49 1.67 2.21 3.1],[3.193 2.2763 1.7201 1.5347 1.7201 2.2763 3.193;2.0909 1.1742 0.7107 0.4326 0.7107 1.1742 2.0909;1.7304 0.8034 0.2472 0.0618 0.2472 0.8034 1.7304;2.0909 1.1742 0.7107 0.4326 0.7107 1.1742 2.0909;3.193 2.2763 1.7201 1.5347 1.7201 2.2763 3.193])  x_losses_mat_4d=cat(4,cat(3,[1.5645 0.441 0.063 0.441 1.5645;1.7535 0.7245 0.252 0.7245 1.7535;2.3205 1.197 0.819 1.197 2.3205;3.255 2.1315 1.764 2.1315 3.255],[1.5645 0.441 0.063 0.441 1.5645;1.7535 0.7245 0.252 0.7245 1.7535;2.3205 1.197 0.819 1.197 2.3205;3.255 2.1315 1.764 2.1315 3.255],[1.5645 0.441 0.063 0.441 1.5645;1.7535 0.7245 0.252 0.7245 1.7535;2.3205 1.197 0.819 1.197 2.3205;3.255 2.1315 1.764 2.1315 3.255]),cat(3,[1.49 0.42 0.06 0.42 1.49;1.67 0.69 0.24 0.69 1.67;2.21 1.14 0.78 1.14 2.21;3.1 2.03 1.68 2.03 3.1],[1.49 0.42 0.06 0.42 1.49;1.67 0.69 0.24 0.69 1.67;2.21 1.14 0.78 1.14 2.21;3.1 2.03 1.68 2.03 3.1],[1.49 0.42 0.06 0.42 1.49;1.67 0.69 0.24 0.69 1.67;2.21 1.14 0.78 1.14 2.21;3.1 2.03 1.68 2.03 3.1]),cat(3,[1.5347 0.4326 0.0618 0.4326 1.5347;1.7201 0.7107 0.2472 0.7107 1.7201;2.2763 1.1742 0.8034 1.1742 2.2763;3.193 2.0909 1.7304 2.0909 3.193],[1.5347 0.4326 0.0618 0.4326 1.5347;1.7201 0.7107 0.2472 0.7107 1.7201;2.2763 1.1742 0.8034 1.1742 2.2763;3.193 2.0909 1.7304 2.0909 3.193],[1.5347 0.4326 0.0618 0.4326 1.5347;1.7201 0.7107 0.2472 0.7107 1.7201;2.2763 1.1742 0.8034 1.1742 2.2763;3.193 2.0909 1.7304 2.0909 3.193]))  CalLossMapData={}  CalLossWithTempMapData={}  aMode=aMode  RefBlkName='autolibmappedmotor/Mapped Motor'
  Mapped Motor1 : autolibmappedmotor/Mapped Motor  w_Tmax_bp_ext=w_Tmax_bp  Tmax_w_V_ext=Tmax_w_V  w_Tmin_bp_ext=w_Tmin_bp  Tmin_w_V_ext=Tmin_w_V  port_config=Speed  param_by=Tabulated torque-speed envelope  w_t=motorSpeedRadPs  T_t=motorMaxTorqueNm  torque_max=.1  power_max=30  SpreadsheetTqLimitsFileName=MotorCalibrationImportData.xlsx  Tmax_w_V=[0.09 0.09 0.09;0.08 0.08 0.08;0.07 0.07 0.07;0 0 0]  w_Tmax_bp=[ 0 375 750 800 ]  V_Tmax_bp=[500 750 900]  Tmin_w_V=[-0.09 -0.09 -0.09;-0.08 -0.08 -0.08;-0.07 -0.07 -0.07;0 0 0]  w_Tmin_bp=[ 0 375 750 800 ]  V_Tmin_bp=[500 750 900]  Tc=0.02  param_loss=Single efficiency measurement  SpreadsheetLossFileName=MotorCalibrationImportData.xlsx  SpreadsheetEffFileName=MotorCalibrationImportData.xlsx  eff=100  w_eff=375  T_eff=0.08  Piron=0  Pbase=0  w_eff_bp=[-8000 -4000 0 4000 8000]  T_eff_bp=[0 0.03 0.06 0.09]  Temp_eff_bp=[233.15 293.15 373.15]  V_eff_bp=[500 700 900]  losses_table=[1.49 1.67 2.21 3.10; 0.42 0.69 1.14 2.03; 0.06 0.24 0.78 1.68; 0.42 0.69 1.14 2.03; 1.49 1.67 2.21 3.10]  losses_table_3d=cat(3,1.05*[1.49 1.67 2.21 3.10; 0.42 0.69 1.14 2.03; 0.06 0.24 0.78 1.68; 0.42 0.69 1.14 2.03; 1.49 1.67 2.21 3.10],[1.49 1.67 2.21 3.10; 0.42 0.69 1.14 2.03; 0.06 0.24 0.78 1.68; 0.42 0.69 1.14 2.03; 1.49 1.67 2.21 3.10],1.03*[1.49 1.67 2.21 3.10; 0.42 0.69 1.14 2.03; 0.06 0.24 0.78 1.68; 0.42 0.69 1.14 2.03; 1.49 1.67 2.21 3.10])  losses_table_4d=cat(4,cat(3,[1.5645 0.441 0.063 0.441 1.5645;1.7535 0.7245 0.252 0.7245 1.7535;2.3205 1.197 0.819 1.197 2.3205;3.255 2.1315 1.764 2.1315 3.255],[1.5645 0.441 0.063 0.441 1.5645;1.7535 0.7245 0.252 0.7245 1.7535;2.3205 1.197 0.819 1.197 2.3205;3.255 2.1315 1.764 2.1315 3.255],[1.5645 0.441 0.063 0.441 1.5645;1.7535 0.7245 0.252 0.7245 1.7535;2.3205 1.197 0.819 1.197 2.3205;3.255 2.1315 1.764 2.1315 3.255]),cat(3,[1.49 0.42 0.06 0.42 1.49;1.67 0.69 0.24 0.69 1.67;2.21 1.14 0.78 1.14 2.21;3.1 2.03 1.68 2.03 3.1],[1.49 0.42 0.06 0.42 1.49;1.67 0.69 0.24 0.69 1.67;2.21 1.14 0.78 1.14 2.21;3.1 2.03 1.68 2.03 3.1],[1.49 0.42 0.06 0.42 1.49;1.67 0.69 0.24 0.69 1.67;2.21 1.14 0.78 1.14 2.21;3.1 2.03 1.68 2.03 3.1]),cat(3,[1.5347 0.4326 0.0618 0.4326 1.5347;1.7201 0.7107 0.2472 0.7107 1.7201;2.2763 1.1742 0.8034 1.1742 2.2763;3.193 2.0909 1.7304 2.0909 3.193],[1.5347 0.4326 0.0618 0.4326 1.5347;1.7201 0.7107 0.2472 0.7107 1.7201;2.2763 1.1742 0.8034 1.1742 2.2763;3.193 2.0909 1.7304 2.0909 3.193],[1.5347 0.4326 0.0618 0.4326 1.5347;1.7201 0.7107 0.2472 0.7107 1.7201;2.2763 1.1742 0.8034 1.1742 2.2763;3.193 2.0909 1.7304 2.0909 3.193]))  efficiency_table=[95 95 95 95; 95 95 95 95; 95 95 95 95; 95 95 95 95; 95 95 95 95]  efficiency_table_3d=cat(3,90*ones(5,4),95*ones(5,4),92*ones(5,4))  efficiency_table_4d=cat(4,cat(3,90*ones(5,4)',90*ones(5,4)',90*ones(5,4)'),cat(3,95*ones(5,4)',95*ones(5,4)',95*ones(5,4)'),cat(3,92*ones(5,4)',92*ones(5,4)',92*ones(5,4)'))  J=5e-6  b=1e-5  omega_o=0  T_t_extended=[166.666666666667 178.571428571429 192.307692307692 208.333333333333 227.272727272727 250 277.777777777778 312.5 357.142857142857 416.666666666667 500 500 500 500 500 500 500 500 500 500 500 416.666666666667 357.142857142857 312.5 277.777777777778 250 227.272727272727 208.333333333333 192.307692307692 178.571428571429 166.666666666667]  w_t_extended=[-600 -560 -520 -480 -440 -400 -360 -320 -280 -240 -200 -160 -120 -80 -40 0 40 80 120 160 200 240 280 320 360 400 440 480 520 560 600]  KLossIron=0  KLossCopper=0  x_w_eff_vec=[-8000 -4000 0 4000 8000]  x_T_eff_vec=[-0.09 -0.06 -0.03 0 0.03 0.06 0.09]  x_tmp_eff_vec=[233.15 293.15 373.15]  x_V_eff_vec=[500 700 900]  x_losses_mat=[3.1 2.21 1.67 1.49 1.67 2.21 3.1;2.03 1.14 0.69 0.42 0.69 1.14 2.03;1.68 0.78 0.24 0.06 0.24 0.78 1.68;2.03 1.14 0.69 0.42 0.69 1.14 2.03;3.1 2.21 1.67 1.49 1.67 2.21 3.1]  x_losses_mat_3d=cat(3,[3.255 2.3205 1.7535 1.5645 1.7535 2.3205 3.255;2.1315 1.197 0.7245 0.441 0.7245 1.197 2.1315;1.764 0.819 0.252 0.063 0.252 0.819 1.764;2.1315 1.197 0.7245 0.441 0.7245 1.197 2.1315;3.255 2.3205 1.7535 1.5645 1.7535 2.3205 3.255],[3.1 2.21 1.67 1.49 1.67 2.21 3.1;2.03 1.14 0.69 0.42 0.69 1.14 2.03;1.68 0.78 0.24 0.06 0.24 0.78 1.68;2.03 1.14 0.69 0.42 0.69 1.14 2.03;3.1 2.21 1.67 1.49 1.67 2.21 3.1],[3.193 2.2763 1.7201 1.5347 1.7201 2.2763 3.193;2.0909 1.1742 0.7107 0.4326 0.7107 1.1742 2.0909;1.7304 0.8034 0.2472 0.0618 0.2472 0.8034 1.7304;2.0909 1.1742 0.7107 0.4326 0.7107 1.1742 2.0909;3.193 2.2763 1.7201 1.5347 1.7201 2.2763 3.193])  x_losses_mat_4d=cat(4,cat(3,[1.5645 0.441 0.063 0.441 1.5645;1.7535 0.7245 0.252 0.7245 1.7535;2.3205 1.197 0.819 1.197 2.3205;3.255 2.1315 1.764 2.1315 3.255],[1.5645 0.441 0.063 0.441 1.5645;1.7535 0.7245 0.252 0.7245 1.7535;2.3205 1.197 0.819 1.197 2.3205;3.255 2.1315 1.764 2.1315 3.255],[1.5645 0.441 0.063 0.441 1.5645;1.7535 0.7245 0.252 0.7245 1.7535;2.3205 1.197 0.819 1.197 2.3205;3.255 2.1315 1.764 2.1315 3.255]),cat(3,[1.49 0.42 0.06 0.42 1.49;1.67 0.69 0.24 0.69 1.67;2.21 1.14 0.78 1.14 2.21;3.1 2.03 1.68 2.03 3.1],[1.49 0.42 0.06 0.42 1.49;1.67 0.69 0.24 0.69 1.67;2.21 1.14 0.78 1.14 2.21;3.1 2.03 1.68 2.03 3.1],[1.49 0.42 0.06 0.42 1.49;1.67 0.69 0.24 0.69 1.67;2.21 1.14 0.78 1.14 2.21;3.1 2.03 1.68 2.03 3.1]),cat(3,[1.5347 0.4326 0.0618 0.4326 1.5347;1.7201 0.7107 0.2472 0.7107 1.7201;2.2763 1.1742 0.8034 1.1742 2.2763;3.193 2.0909 1.7304 2.0909 3.193],[1.5347 0.4326 0.0618 0.4326 1.5347;1.7201 0.7107 0.2472 0.7107 1.7201;2.2763 1.1742 0.8034 1.1742 2.2763;3.193 2.0909 1.7304 2.0909 3.193],[1.5347 0.4326 0.0618 0.4326 1.5347;1.7201 0.7107 0.2472 0.7107 1.7201;2.2763 1.1742 0.8034 1.1742 2.2763;3.193 2.0909 1.7304 2.0909 3.193]))  CalLossMapData={}  CalLossWithTempMapData={}  aMode=aMode  RefBlkName='autolibmappedmotor/Mapped Motor'
  Mux : Mux  Inputs=2
  Rotational Inertia F : autolibsharedcoupling/Rotational Inertia  port_config=Simulink  extInfo=off  externJ=off  J=.001  b=.001  omega_o=0  blkID=0  aMode=1
      settings: LibrarySourceBlock=autolibcoupling/Rotational Inertia
  Rotational Inertia R : autolibsharedcoupling/Rotational Inertia  port_config=Simulink  extInfo=off  externJ=off  J=.001  b=.001  omega_o=0  blkID=0  aMode=1
      settings: LibrarySourceBlock=autolibcoupling/Rotational Inertia
  Scope : Scope
  Sum : Sum  Inputs=|++
  Transfer Fcn : TransferFcn  Denominator=[0.01 1]
  Transfer Fcn1 : TransferFcn  Denominator=[0.01 1]
  Two-Way Connection1 : TwoWayConnection
  Two-Way Connection5 : TwoWayConnection
  M1 : PMIOPort  Side=Right
  M2 : PMIOPort  Port=2  Side=Right
  MotSpd : Outport
  SOC : Outport  Port=2
  Mot2Spd : Outport  Port=3
  tag scope: Te_actual=global
  wires:
  Rotational Inertia F/1 -> Mapped Motor/2, MotSpd/1, Two-Way Connection5/1
  Datasheet Battery/2 -> Scope/1
  Mapped Motor/3 -> Mux/1, Rotational Inertia F/1
  TrqMCUCmd_F/1 -> Mapped Motor/3
  Two-Way Connection5/1 -> Rotational Inertia F/2
  Constant2/1 -> Datasheet Battery/2
  Mapped Motor/2 -> Transfer Fcn/1  "BattCurr"
  Datasheet Battery/1 -> Bus Selector/1
  Bus Selector/1 -> Gain/1  "<BattSoc>"
  Gain/1 -> SOC/1
  Rotational Inertia R/1 -> Mapped Motor1/2, Mot2Spd/1, Two-Way Connection1/1
  Mapped Motor1/3 -> Mux/2, Rotational Inertia R/1
  Two-Way Connection1/1 -> Rotational Inertia R/2
  TrqMCUCmd_R/1 -> Mapped Motor1/3
  Mapped Motor1/2 -> Transfer Fcn1/1  "BattCurr"
  Transfer Fcn/1 -> Sum/1
  Transfer Fcn1/1 -> Sum/2
  Sum/1 -> Datasheet Battery/1
  Mux/1 -> [Te_actual]
  Constant/1 -> Mapped Motor1/1, Mapped Motor/1
  connections:
  Two-Way Connection5/RConn1 -- M1/RConn1
  Two-Way Connection1/RConn1 -- M2/RConn1

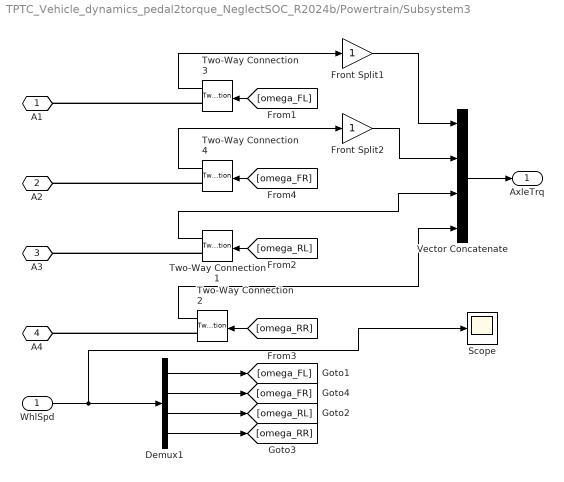
== system TPTC_Vehicle_dynamics_pedal2torque_NeglectSOC_R2024b/Powertrain/Subsystem3 ==
  WhlSpd : Inport
  Demux1 : Demux
  Front Split1 : Gain
  Front Split2 : Gain
  Scope : Scope
  Two-Way Connection{1..4} (4 alike) : TwoWayConnection
  Vector Concatenate : Concatenate  NumInputs=4
  A1 : PMIOPort  Side=Left
  A2 : PMIOPort  Port=2  Side=Left
  A3 : PMIOPort  Port=3  Side=Left
  A4 : PMIOPort  Port=4  Side=Left
  AxleTrq : Outport  VectorParamsAs1DForOutWhenUnconnected=off
  wires:
  Two-Way Connection1/1 -> Vector Concatenate/3
  Front Split1/1 -> Vector Concatenate/1
  [omega_RL] -> Two-Way Connection1/1
  Demux1/4 -> [omega_RR]
  Demux1/1 -> [omega_FL]
  Demux1/2 -> [omega_FR]
  Vector Concatenate/1 -> AxleTrq/1
  Demux1/3 -> [omega_RL]
  [omega_FL] -> Two-Way Connection3/1
  [omega_FR] -> Two-Way Connection4/1
  Front Split2/1 -> Vector Concatenate/2
  [omega_RR] -> Two-Way Connection2/1
  Two-Way Connection3/1 -> Front Split1/1
  Two-Way Connection2/1 -> Vector Concatenate/4
  WhlSpd/1 -> Scope/1, Demux1/1
  Two-Way Connection4/1 -> Front Split2/1
  connections:
  Two-Way Connection3/RConn1 -- A1/RConn1
  Two-Way Connection2/RConn1 -- A4/RConn1
  Two-Way Connection1/RConn1 -- A3/RConn1
  Two-Way Connection4/RConn1 -- A2/RConn1

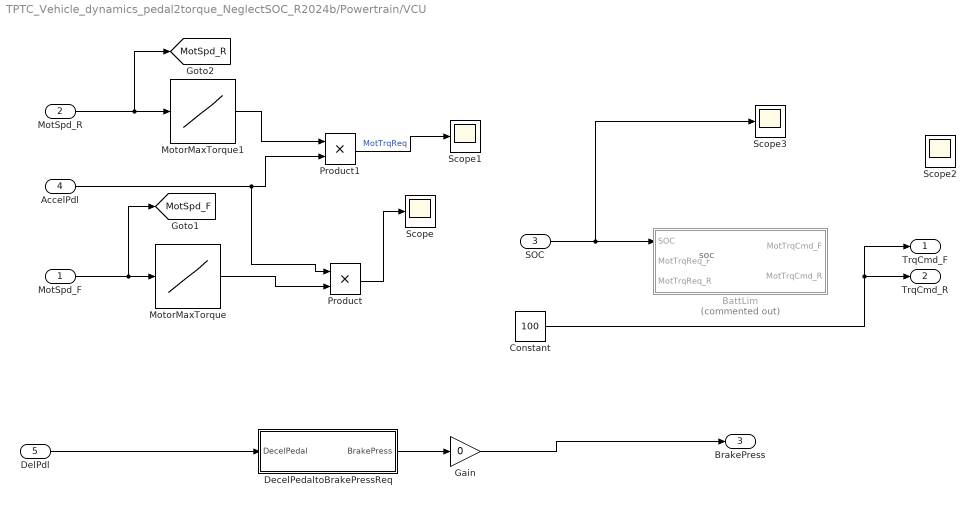
== system TPTC_Vehicle_dynamics_pedal2torque_NeglectSOC_R2024b/Powertrain/VCU ==
  note: soc
  MotSpd_F : Inport
  MotSpd_R : Inport  Port=2
  SOC : Inport  Port=3
  AccelPdl : Inport  Port=4
  DelPdl : Inport  Port=5
  BattLim : Subsystem  Commented=on
  Constant : Constant  Value=100
  DecelPedaltoBrakePressReq : Subsystem
  Gain : Gain  Gain=0
  MotorMaxTorque : Lookup_n-D  NumberOfTableDimensions=1  BreakpointsForDimension1=motorSpeedRadPs  Table=motorMaxTorqueNm  ExtrapMethod=Clip  InternalRulePriority=Speed  RndMeth=Simplest
  MotorMaxTorque1 : Lookup_n-D  NumberOfTableDimensions=1  BreakpointsForDimension1=motorSpeedRadPs  Table=motorMaxTorqueNm  ExtrapMethod=Clip  InternalRulePriority=Speed  RndMeth=Simplest
  Product : Product
  Product1 : Product
  Scope{,1..3} (4 alike) : Scope
  TrqCmd_F : Outport
  TrqCmd_R : Outport  Port=2
  BrakePress : Outport  Port=3
  tag scope: MotSpd_F=global, MotSpd_R=global
  wires:
  DelPdl/1 -> DecelPedaltoBrakePressReq/1(DecelPedal)
  Product/1 -> Scope/1
  MotSpd_F/1 -> MotorMaxTorque/1, [MotSpd_F]
  SOC/1 -> Scope3/1, BattLim/1(SOC)
  DecelPedaltoBrakePressReq/1(BrakePress) -> Gain/1
  MotSpd_R/1 -> [MotSpd_R], MotorMaxTorque1/1
  MotorMaxTorque1/1 -> Product1/1
  Gain/1 -> BrakePress/1
  AccelPdl/1 -> Product/1, Product1/2
  Product1/1 -> Scope1/1  "MotTrqReq"
  MotorMaxTorque/1 -> Product/2
  Constant/1 -> TrqCmd_R/1, TrqCmd_F/1

== system TPTC_Vehicle_dynamics_pedal2torque_NeglectSOC_R2024b/Environment/Ground Feedback/Constant ==
  Friction : Inport
  Bus Creator : BusCreator  Inputs=4
  Bus Creator2 : BusCreator  Inputs=4
  Bus Creator3 : BusCreator  Inputs=3
  Constant1 : Constant  Value=zeros(4,1)
  Constant2 : Constant  Value=repmat(eye(3),1,1,4)  SampleTime=-1
  Demux : Demux
  Demux1 : Demux
  Signal Specification : SignalSpecification  Unit=m
  Signal Specification1 : SignalSpecification  Unit=1
  Ground : Outport  VectorParamsAs1DForOutWhenUnconnected=off
  wires:
  Constant1/1 -> Signal Specification/1
  Signal Specification/1 -> Demux/1
  Demux/4 -> Bus Creator/4  "G_RR_z"
  Demux/1 -> Bus Creator/1  "G_FL_z"
  Demux/3 -> Bus Creator/3  "G_RL_z"
  Demux/2 -> Bus Creator/2  "G_FR_z"
  Bus Creator/1 -> Bus Creator3/1  "z"
  Demux1/3 -> Bus Creator2/3  "mu_RL"
  Demux1/4 -> Bus Creator2/4  "mu_RR"
  Demux1/1 -> Bus Creator2/1  "mu_FL"
  Demux1/2 -> Bus Creator2/2  "mu_FR"
  Bus Creator2/1 -> Bus Creator3/3  "mu"
  Friction/1 -> Signal Specification1/1
  Signal Specification1/1 -> Demux1/1
  Bus Creator3/1 -> Ground/1
  Constant2/1 -> Bus Creator3/2  "DCM"

== system TPTC_Vehicle_dynamics_pedal2torque_NeglectSOC_R2024b/Powertrain/03_MCU_TPTC_Controller/Command_Merge_Front ==
  T_vcu : Inport
  Tlim : Inport  Port=2
  T_damp : Inport  Port=3
  Demux1 : Demux  Outputs=2
  Demux2 : Demux  Outputs=2
  Demux3 : Demux  Outputs=2
  Fast_Down_Slow_Up_Limiter : MATLAB Function  TreatAsAtomicUnit=on
  Scope : Scope  NumInputPorts=3
  MT_vcu_f : Outport
  MT_vcu_r : Outport  Port=2
  wires:
  Fast_Down_Slow_Up_Limiter/2(T_cmd_r) -> Scope/2, MT_vcu_r/1
  Fast_Down_Slow_Up_Limiter/1(T_cmd_f) -> Scope/1, MT_vcu_f/1
  Demux1/1 -> Fast_Down_Slow_Up_Limiter/1(T_vcu_f)
  Demux1/2 -> Fast_Down_Slow_Up_Limiter/2(T_vcu_r)
  Tlim/1 -> Demux2/1
  Demux2/1 -> Fast_Down_Slow_Up_Limiter/3(Tlim_f)
  Demux2/2 -> Fast_Down_Slow_Up_Limiter/4(Tlim_r)
  T_damp/1 -> Demux3/1
  Demux3/1 -> Fast_Down_Slow_Up_Limiter/5(T_damp_f)
  Demux3/2 -> Fast_Down_Slow_Up_Limiter/6(T_damp_r)
  T_vcu/1 -> Scope/3, Demux1/1

== system TPTC_Vehicle_dynamics_pedal2torque_NeglectSOC_R2024b/Powertrain/03_MCU_TPTC_Controller/Load_Observer ==
  Te_hat_F : Inport
  alpha_motor_F : Inport  Port=2
  Te_hat_R : Inport  Port=3
  alpha_motor_R : Inport  Port=4
  J_eq_motor : Gain  Gain=J_axle
  J_eq_motor1 : Gain  Gain=J_axle
  Saturation_nonnegative : Saturate  UpperLimit=Tmax_mot  LowerLimit=0
  Saturation_nonnegative1 : Saturate  UpperLimit=Tmax_mot  LowerLimit=0
  Scope1 : Scope
  Scope2 : Scope
  Scope3 : Scope
  Te_minus_Jalpha : Sum  Inputs=+-
  Te_minus_Jalpha1 : Sum  Inputs=+-
  Tload_hat_F : Outport
  Tload_hat_R : Outport  Port=2
  wires:
  alpha_motor_F/1 -> Scope3/1, J_eq_motor/1
  Te_hat_F/1 -> Te_minus_Jalpha/1
  J_eq_motor/1 -> Scope2/1, Te_minus_Jalpha/2
  Te_minus_Jalpha/1 -> Scope1/1, Saturation_nonnegative/1
  Saturation_nonnegative/1 -> Tload_hat_F/1
  Te_hat_R/1 -> Te_minus_Jalpha1/1
  Saturation_nonnegative1/1 -> Tload_hat_R/1
  J_eq_motor1/1 -> Te_minus_Jalpha1/2
  alpha_motor_R/1 -> J_eq_motor1/1
  Te_minus_Jalpha1/1 -> Saturation_nonnegative1/1

== system TPTC_Vehicle_dynamics_pedal2torque_NeglectSOC_R2024b/Powertrain/03_MCU_TPTC_Controller/Motor_Acceleration_Estimation ==
  omega_m_f : Inport
  omega_m_r : Inport  Port=2
  Discrete Transfer Fcn : DiscreteTransferFcn  LoadFcn=dspblkCoreblockFVToolHelper(gcbh,'load');  Numerator=[0.0487706]  Denominator=[1 -0.951229]
      settings: CopyFcn=dspblkCoreblockFVToolHelper(gcbh,'copy');  DeleteFcn=dspblkCoreblockFVToolHelper(gcbh,'close');  ModelCloseFcn=dspblkCoreblockFVToolHelper(gcbh,'close');  PreSaveFcn=dspblkCoreblockFVToolHelper(gcbh,'presave');  PostSaveFcn=dspblkCoreblockFVToolHelper(gcbh,'postsave');  CloseFcn=dspblkCoreblockFVToolHelper(gcbh,'close');
  Discrete Transfer Fcn1 : DiscreteTransferFcn  LoadFcn=dspblkCoreblockFVToolHelper(gcbh,'load');  Numerator=[0.0487706]  Denominator=[1 -0.951229]
      settings: CopyFcn=dspblkCoreblockFVToolHelper(gcbh,'copy');  DeleteFcn=dspblkCoreblockFVToolHelper(gcbh,'close');  ModelCloseFcn=dspblkCoreblockFVToolHelper(gcbh,'close');  PreSaveFcn=dspblkCoreblockFVToolHelper(gcbh,'presave');  PostSaveFcn=dspblkCoreblockFVToolHelper(gcbh,'postsave');  CloseFcn=dspblkCoreblockFVToolHelper(gcbh,'close');
  Gain : Gain  Gain=1/Ts_asr
  Gain1 : Gain  Gain=1/Ts_asr
  Sum : Sum  Inputs=|+-
  Sum1 : Sum  Inputs=|+-
  Unit Delay : UnitDelay  SampleTime=-1
  Unit Delay1 : UnitDelay  SampleTime=-1
  alpha_m_f : Outport
  alpha_m_r : Outport  Port=2
  wires:
  omega_m_f/1 -> Sum/1, Unit Delay/1
  Unit Delay/1 -> Sum/2
  Sum/1 -> Gain/1
  Gain/1 -> Discrete Transfer Fcn/1
  Discrete Transfer Fcn/1 -> alpha_m_f/1
  Gain1/1 -> Discrete Transfer Fcn1/1
  omega_m_r/1 -> Sum1/1, Unit Delay1/1
  Sum1/1 -> Gain1/1
  Unit Delay1/1 -> Sum1/2
  Discrete Transfer Fcn1/1 -> alpha_m_r/1

== system TPTC_Vehicle_dynamics_pedal2torque_NeglectSOC_R2024b/Powertrain/03_MCU_TPTC_Controller/ReaL_Load_Force ==
  Add1 : Sum
  Add2 : Sum
  Demux : Demux
  Demux1 : Demux
  F to Torque : Gain  Gain=R_tire *1 / (gear_ratio_R * eta_drv);
  F to Torque1 : Gain  Gain=R_tire *1 / (gear_ratio_F * eta_drv);
  ReaL_Load_Force_Front : Outport
  ReaL_Load_Force_Rear : Outport  Port=2
  wires:
  Demux1/2 -> Add2/2
  F to Torque/1 -> Demux/1
  [Fx] -> F to Torque1/1
  [Fx] -> F to Torque/1
  F to Torque1/1 -> Demux1/1
  Demux/4 -> Add1/2
  Demux/3 -> Add1/1
  Demux1/1 -> Add2/1
  Add2/1 -> ReaL_Load_Force_Front/1
  Add1/1 -> ReaL_Load_Force_Rear/1

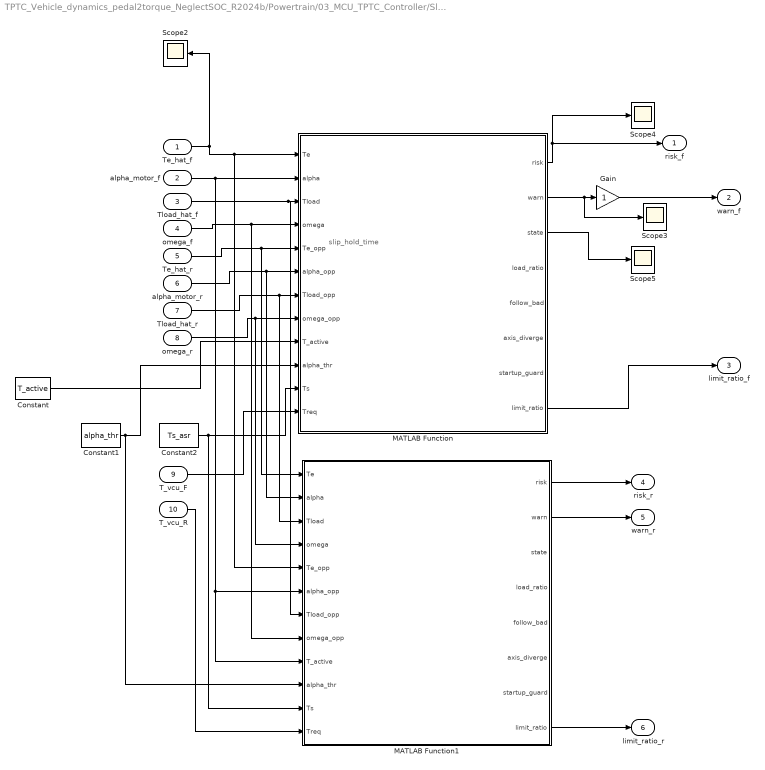
== system TPTC_Vehicle_dynamics_pedal2torque_NeglectSOC_R2024b/Powertrain/03_MCU_TPTC_Controller/Slip_Detector_Front ==
  note: slip_hold_time
  Te_hat_f : Inport
  alpha_motor_f : Inport  Port=2
  Tload_hat_f : Inport  Port=3
  omega_f : Inport  Port=4
  Te_hat_r : Inport  Port=5
  alpha_motor_r : Inport  Port=6
  Tload_hat_r : Inport  Port=7
  omega_r : Inport  Port=8
  T_vcu_F : Inport  Port=9
  T_vcu_R : Inport  Port=10
  Constant : Constant  Value=T_active
  Constant1 : Constant  Value=alpha_thr
  Constant2 : Constant  Value=Ts_asr
  Gain : Gain
  MATLAB Function : MATLAB Function  TreatAsAtomicUnit=on  SystemSampleTime=Ts_asr
  MATLAB Function1 : MATLAB Function  TreatAsAtomicUnit=on  SystemSampleTime=Ts_asr
  Scope{2..5} (4 alike) : Scope
  risk_f : Outport
  warn_f : Outport  Port=2
  limit_ratio_f : Outport  Port=3
  risk_r : Outport  Port=4
  warn_r : Outport  Port=5
  limit_ratio_r : Outport  Port=6
  wires:
  Tload_hat_f/1 -> MATLAB Function1/7(Tload_opp), MATLAB Function/3(Tload)
  alpha_motor_f/1 -> MATLAB Function1/9(T_active), MATLAB Function1/6(alpha_opp), MATLAB Function/2(alpha)
  Te_hat_f/1 -> Scope2/1, MATLAB Function1/5(Te_opp), MATLAB Function/1(Te)
  MATLAB Function/1(risk) -> Scope4/1, risk_f/1
  MATLAB Function/2(warn) -> Scope3/1, Gain/1
  MATLAB Function/3(state) -> Scope5/1
  Gain/1 -> warn_f/1
  omega_f/1 -> MATLAB Function1/8(omega_opp), MATLAB Function/4(omega)
  alpha_motor_r/1 -> MATLAB Function1/2(alpha), MATLAB Function/6(alpha_opp)
  Tload_hat_r/1 -> MATLAB Function1/3(Tload), MATLAB Function/7(Tload_opp)
  omega_r/1 -> MATLAB Function1/4(omega), MATLAB Function/8(omega_opp)
  Constant/1 -> MATLAB Function/9(T_active)
  Constant1/1 -> MATLAB Function/10(alpha_thr), MATLAB Function1/10(alpha_thr)
  Constant2/1 -> MATLAB Function1/11(Ts), MATLAB Function/11(Ts)
  T_vcu_F/1 -> MATLAB Function/12(Treq)
  MATLAB Function/8(limit_ratio) -> limit_ratio_f/1
  Te_hat_r/1 -> MATLAB Function1/1(Te), MATLAB Function/5(Te_opp)
  MATLAB Function1/8(limit_ratio) -> limit_ratio_r/1
  MATLAB Function1/1(risk) -> risk_r/1
  MATLAB Function1/2(warn) -> warn_r/1
  T_vcu_R/1 -> MATLAB Function1/12(Treq)

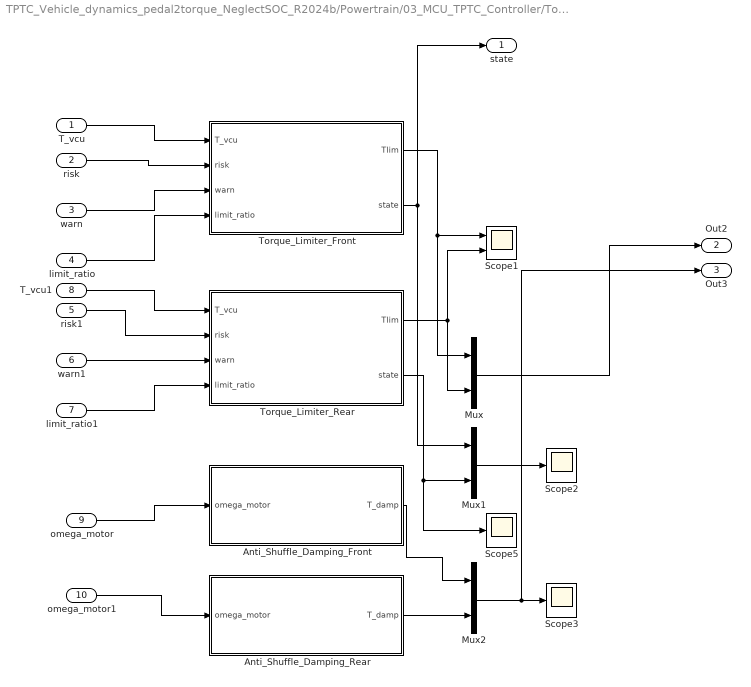
== system TPTC_Vehicle_dynamics_pedal2torque_NeglectSOC_R2024b/Powertrain/03_MCU_TPTC_Controller/Torque_Limiter ==
  T_vcu : Inport
  risk : Inport  Port=2
  warn : Inport  Port=3
  limit_ratio : Inport  Port=4
  risk1 : Inport  Port=5
  warn1 : Inport  Port=6
  limit_ratio1 : Inport  Port=7
  T_vcu1 : Inport  Port=8
  omega_motor : Inport  Port=9
  omega_motor1 : Inport  Port=10
  Anti_Shuffle_Damping_Front : Subsystem
  Anti_Shuffle_Damping_Rear : Subsystem
  Mux : Mux  Inputs=2
  Mux1 : Mux  Inputs=2
  Mux2 : Mux  Inputs=2
  Scope1 : Scope  NumInputPorts=2
  Scope2 : Scope
  Scope3 : Scope
  Scope5 : Scope
  Torque_Limiter_Front : Subsystem
  Torque_Limiter_Rear : Subsystem
  state : Outport
  Out2 : Outport  Port=2
  Out3 : Outport  Port=3
  wires:
  omega_motor1/1 -> Anti_Shuffle_Damping_Rear/1(omega_motor)
  Mux2/1 -> Out3/1, Scope3/1
  Torque_Limiter_Rear/2(state) -> Scope5/1, Mux1/2
  Anti_Shuffle_Damping_Front/1(T_damp) -> Mux2/1
  Anti_Shuffle_Damping_Rear/1(T_damp) -> Mux2/2
  risk1/1 -> Torque_Limiter_Rear/2(risk)
  Torque_Limiter_Rear/1(Tlim) -> Scope1/2, Mux/2
  Mux1/1 -> Scope2/1
  Torque_Limiter_Front/1(Tlim) -> Scope1/1, Mux/1
  Torque_Limiter_Front/2(state) -> state/1, Mux1/1
  T_vcu1/1 -> Torque_Limiter_Rear/1(T_vcu)
  limit_ratio/1 -> Torque_Limiter_Front/4(limit_ratio)
  risk/1 -> Torque_Limiter_Front/2(risk)
  warn/1 -> Torque_Limiter_Front/3(warn)
  omega_motor/1 -> Anti_Shuffle_Damping_Front/1(omega_motor)
  limit_ratio1/1 -> Torque_Limiter_Rear/4(limit_ratio)
  Mux/1 -> Out2/1
  warn1/1 -> Torque_Limiter_Rear/3(warn)
  T_vcu/1 -> Torque_Limiter_Front/1(T_vcu)
